simulink model "SMC_controller"  (R2025a)
settings: Solver=VariableStepAuto  StartTime=0.0  StopTime=t_total(end)  RelTol=1e-3
StopFcn:
  | autoplot;
values from neighbouring files (symbols this model uses):
  Ib = diag([params.Ix, params.Iy, params.Iz])    [setup_mission.m]
  lin_vel_0 = [0; 0; 0]    [setup_mission.m]
  mass = params.m    [setup_mission.m]
  pos_0 = p_ref(:,1) + offset_init    [setup_mission.m]
  w_bb_0 = [0; 0; 0]    [setup_mission.m]
libraries: robotcorelib x2, uavutilslib x1
settings Model: Creator=marco  LastModifiedBy=marco

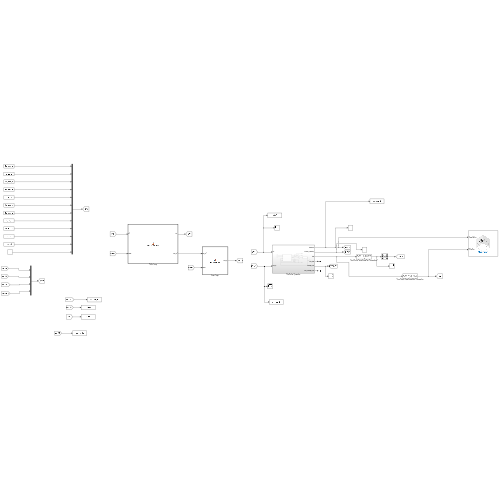
[thumbnail: Simulink's stored preview of the top-level diagram]
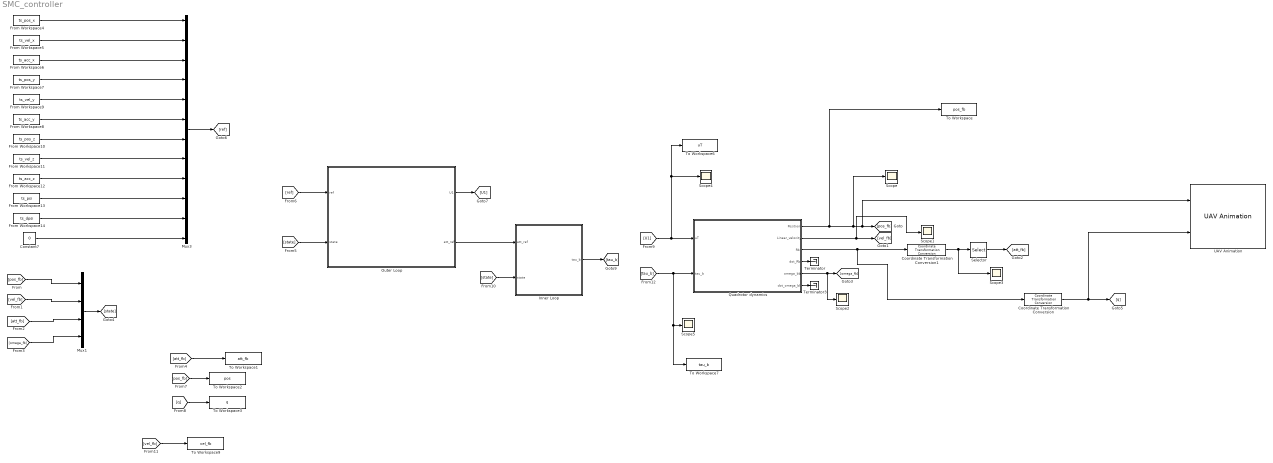
== system SMC_controller ==
  Constant7 : Constant  Value=0
  Coordinate Transformation Conversion : robotcorelib/Coordinate Transformation Conversion  InputRepresentation=Rotation Matrix  InputEulerSequence=ZYX  ShowTrVecInputPort=on  OutputRepresentation=Quaternion  OutputEulerSequence=ZYX  ShowTrVecOutputPort=on  SimulateUsing=Interpreted execution
  Coordinate Transformation Conversion1 : robotcorelib/Coordinate Transformation Conversion  InputRepresentation=Rotation Matrix  InputEulerSequence=ZYX  ShowTrVecInputPort=on  OutputRepresentation=Euler Angles  OutputEulerSequence=ZYX  ShowTrVecOutputPort=on  SimulateUsing=Interpreted execution
  From Workspace10 : FromWorkspace  VariableName=ts_pos_z
  From Workspace11 : FromWorkspace  VariableName=ts_vel_z
  From Workspace12 : FromWorkspace  VariableName=ts_acc_z
  From Workspace13 : FromWorkspace  VariableName=ts_psi
  From Workspace14 : FromWorkspace  VariableName=ts_dpsi
  From Workspace4 : FromWorkspace  VariableName=ts_pos_x
  From Workspace5 : FromWorkspace  VariableName=ts_vel_x
  From Workspace6 : FromWorkspace  VariableName=ts_acc_x
  From Workspace7 : FromWorkspace  VariableName=ts_pos_y
  From Workspace8 : FromWorkspace  VariableName=ts_acc_y
  From Workspace9 : FromWorkspace  VariableName=ts_vel_y
  Inner Loop : MATLAB Function  TreatAsAtomicUnit=on
  Mux1 : Mux
  Mux3 : Mux  Inputs=12
  Outer Loop : MATLAB Function  TreatAsAtomicUnit=on
  Quadrotor dynamics : Subsystem
  Scope{,1..5} (6 alike) : Scope
      Scope settings: ActiveDisplayYMinimum=-3.15015245464377  ActiveDisplayYMaximum=14.919654121534494
      Scope1 settings: ActiveDisplayYMinimum=-2.7455147256808767  ActiveDisplayYMaximum=2.7455147553704635
      Scope2 settings: ActiveDisplayYMinimum=-1  ActiveDisplayYMaximum=1  DataLoggingVariableName=ScopeData2
      Scope3 settings: ActiveDisplayYMinimum=-1  ActiveDisplayYMaximum=1  DataLoggingVariableName=ScopeData3
      Scope4 settings: ActiveDisplayYMinimum=4.05773159000642  ActiveDisplayYMaximum=6.8393308416800735  DataLoggingVariableName=ScopeData4
      Scope5 settings: ActiveDisplayYMinimum=-0.047587391271412371  ActiveDisplayYMaximum=0.017818503987418778  DataLoggingVariableName=ScopeData5
  Selector : Selector  InputPortWidth=3  IndexOptions=Index vector (dialog)  Indices=[3, 2, 1]  OutputSizes=1
  Terminator : Terminator
  Terminator3 : Terminator
  To Workspace : ToWorkspace  VariableName=pos_fb  SaveFormat=Timeseries  SampleTime=-1
  To Workspace1 : ToWorkspace  VariableName=att_fb  SaveFormat=Timeseries  SampleTime=-1
  To Workspace2 : ToWorkspace  VariableName=pos  SaveFormat=Timeseries  SampleTime=-1
  To Workspace3 : ToWorkspace  VariableName=q  SaveFormat=Timeseries  SampleTime=-1
  To Workspace6 : ToWorkspace  VariableName=uT  SaveFormat=Timeseries  SampleTime=-1
  To Workspace7 : ToWorkspace  VariableName=tau_b  SaveFormat=Timeseries  SampleTime=-1
  To Workspace9 : ToWorkspace  VariableName=vel_fb  SaveFormat=Timeseries  SampleTime=-1
  UAV Animation : uavutilslib/UAV Animation  NumUAV=1  DynamicUAVConfig=off  UAVType=Multirotor  UAVSize=1  UAVColor=[1 0 0]  UAVTrajectoryAlpha=1  InertialZDirection=Down  RotationFormat=Quaternion  DrawMarkers=off  SampleTime=0.01
  wires:
  [att_fb] -> Mux1/3
  [pos_fb] -> Mux1/1
  Selector/1 -> [att_fb]
  [omega_fb] -> Mux1/4
  Coordinate Transformation Conversion1/1 -> Selector/1, Scope3/1
  Quadrotor dynamics/3(Rb) -> Coordinate Transformation Conversion/1, Coordinate Transformation Conversion1/1
  Quadrotor dynamics/2(Linear_velocity) -> Scope1/1, [vel_fb]
  Quadrotor dynamics/1(Position) -> To Workspace/1, Scope/1, UAV Animation/1, [pos_fb]
  Quadrotor dynamics/5(omega_bb) -> Scope2/1, [omega_fb]
  Coordinate Transformation Conversion/1 -> UAV Animation/2, [q]
  [vel_fb] -> Mux1/2
  Quadrotor dynamics/4(dot_Rb) -> Terminator/1
  Quadrotor dynamics/6(dot_omega_bb) -> Terminator3/1
  [att_fb] -> To Workspace1/1
  Mux1/1 -> [state]
  Mux3/1 -> [ref]
  From Workspace6/1 -> Mux3/3
  From Workspace5/1 -> Mux3/2
  From Workspace4/1 -> Mux3/1
  From Workspace7/1 -> Mux3/4
  From Workspace9/1 -> Mux3/5
  From Workspace8/1 -> Mux3/6
  From Workspace10/1 -> Mux3/7
  From Workspace11/1 -> Mux3/8
  From Workspace12/1 -> Mux3/9
  From Workspace13/1 -> Mux3/10
  Constant7/1 -> Mux3/12
  From Workspace14/1 -> Mux3/11
  [pos_fb] -> To Workspace2/1
  [q] -> To Workspace3/1
  [vel_fb] -> To Workspace9/1
  [state] -> Inner Loop/2(state)
  Inner Loop/1(tau_b) -> [tau_b]
  Outer Loop/2(att_ref) -> Inner Loop/1(att_ref)
  Outer Loop/1(U1) -> [U1]
  [state] -> Outer Loop/2(state)
  [ref] -> Outer Loop/1(ref)
  [U1] -> Scope4/1, To Workspace6/1, Quadrotor dynamics/1(uT)
  [tau_b] -> To Workspace7/1, Scope5/1, Quadrotor dynamics/2(tau_b)

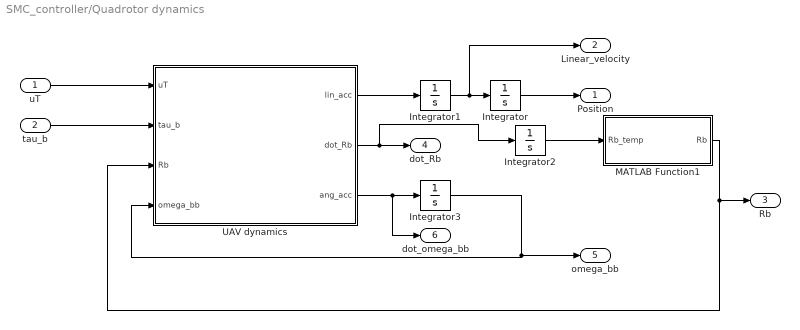
== system SMC_controller/Quadrotor dynamics ==
  uT : Inport
  tau_b : Inport  Port=2
  Integrator : Integrator  InitialCondition=pos_0
  Integrator1 : Integrator  InitialCondition=lin_vel_0
  Integrator2 : Integrator  InitialCondition=[1 0 0; 0 1 0;0 0 1]
  Integrator3 : Integrator  InitialCondition=w_bb_0
  MATLAB Function1 : MATLAB Function  TreatAsAtomicUnit=on
  UAV dynamics : MATLAB Function  TreatAsAtomicUnit=on
  Position : Outport
  Linear_velocity : Outport  Port=2
  Rb : Outport  Port=3
  dot_Rb : Outport  Port=4
  omega_bb : Outport  Port=5
  dot_omega_bb : Outport  Port=6
  wires:
  tau_b/1 -> UAV dynamics/2(tau_b)
  Integrator/1 -> Position/1
  UAV dynamics/3(ang_acc) -> dot_omega_bb/1, Integrator3/1
  UAV dynamics/1(lin_acc) -> Integrator1/1
  uT/1 -> UAV dynamics/1(uT)
  Integrator1/1 -> Linear_velocity/1, Integrator/1
  Integrator3/1 -> UAV dynamics/4(omega_bb), omega_bb/1
  UAV dynamics/2(dot_Rb) -> Integrator2/1, dot_Rb/1
  MATLAB Function1/1(Rb) -> Rb/1, UAV dynamics/3(Rb)
  Integrator2/1 -> MATLAB Function1/1(Rb_temp)

== matlab function SMC_controller/Quadrotor dynamics/UAV dynamics ==
  data: uT input size=1; tau_b input size=3; lin_acc output size=3; Rb input size=[3,3]; omega_bb input size=3; dot_Rb output size=[3,3]; ang_acc output size=3; mass parameter size=1; Ib parameter size=[3,3]
function [lin_acc, dot_Rb, ang_acc] = fcn(uT,tau_b,Rb,omega_bb,mass, Ib)

lin_acc = 9.81*[0 0 1]'-(uT/mass)*Rb*[0 0 1]';
dot_Rb = Rb*skew(omega_bb);
ang_acc = inv(Ib)*(-skew(omega_bb)*Ib*omega_bb + tau_b);

end

function S = skew(v)
if(numel(v)~= 1)
S= [0 -v(3) v(2); 
    v(3) 0 -v(1);
    -v(2) v(1) 0];
else
S= zeros(3);
end
end

== matlab function SMC_controller/Outer Loop ==
  data: ref input; U1 output; state input; att_ref output; params parameter
function [U1, att_ref] = smc_outer_loop(ref, state, params)
% --- SMC OUTER LOOP (POSIZIONE) ---

%% 1. ESTRAZIONE DATI
x = state(1); y = state(2); z = state(3);
vx = state(4); vy = state(5); vz = state(6);
psi = state(9); % Serve per estrarre gli angoli desiderati

xd = ref(1); vxd = ref(2); axd = ref(3);
yd = ref(4); vyd = ref(5); ayd = ref(6);
zd = ref(7); vzd = ref(8); azd = ref(9);
psid = ref(10); dpsid = ref(11);

m = params.m; g = params.g;

%% 2. PARAMETRI DI TUNING (Posizione)
lam_x = 4.0;  K_x = 5.0;   
lam_y = 4.0;  K_y = 3.0;   
lam_z = 5.0;  K_z = 12.0;  
sat_width = 0.5; 

%% 3. CONTROLLO POSIZIONE
ex = xd - x;  edot_x = vxd - vx;
ey = yd - y;  edot_y = vyd - vy;
ez = zd - z;  edot_z = vzd - vz;

Sx = edot_x + lam_x * ex;
Sy = edot_y + lam_y * ey;
Sz = edot_z + lam_z * ez;

Ux = axd + lam_x * edot_x + K_x * tanh(Sx / sat_width);
Uy = ayd + lam_y * edot_y + K_y * tanh(Sy / sat_width);
Uz = azd + lam_z * edot_z + K_z * tanh(Sz / sat_width);

% --- Calcolo U1 (Thrust) ---
total_acc_z = g - Uz; 
U1 = m * sqrt(Ux^2 + Uy^2 + total_acc_z^2);

% Safety Clamp
if U1 > 20 * m * g
    U1 = 20 * m * g; 
end

% --- CALCOLO ANGOLI (FIXED) ---
phi_d_raw   = (Uy * cos(psi) - Ux * sin(psi)) / g; 
theta_d_raw = -1 * (Ux * cos(psi) + Uy * sin(psi)) / g;

phi_d   = max(-0.5, min(0.5, phi_d_raw));
theta_d = max(-0.5, min(0.5, theta_d_raw));

%% 4. OUTPUT VERSO L'INNER LOOP
% Pacchettizziamo i riferimenti di attitudine da passare all'Inner Loop
att_ref = [phi_d; theta_d; psid; dpsid];

end

== matlab function SMC_controller/Inner Loop ==
  data: att_ref input; tau_b output; state input; params parameter
function tau_b  = smc_inner_loop(att_ref, state, params)
% --- SMC INNER LOOP (ATTITUDINE) ---

%% 1. ESTRAZIONE DATI
% Estrazione riferimenti dall'Outer Loop
phi_d = att_ref(1); 
theta_d = att_ref(2);
psid = att_ref(3); 
dpsid = att_ref(4);

phi = state(7); theta = state(8); psi = state(9);
p = state(10); q = state(11); r = state(12);

Ix = params.Ix; Iy = params.Iy; Iz = params.Iz;

%% 2. PARAMETRI DI TUNING (Attitudine)
lam_phi = 15.0;   K_phi = 25.0; 
lam_theta = 15.0; K_theta = 25.0;
lam_psi = 8.0;    K_psi = 10.0;
sat_width = 0.5; 

%% 3. CONTROLLO ATTITUDINE
e_phi   = phi_d - phi;
e_theta = theta_d - theta;
e_psi   = psid - psi;

edot_phi   = 0 - p; 
edot_theta = 0 - q; 
edot_psi   = dpsid - r; 

S_phi   = edot_phi   + lam_phi   * e_phi;
S_theta = edot_theta + lam_theta * e_theta;
S_psi   = edot_psi   + lam_psi   * e_psi;

% --- COPPIE STANDARD ---
U2 = Ix * (lam_phi   * edot_phi   + K_phi   * tanh(S_phi   / sat_width));
U3 = Iy * (lam_theta * edot_theta + K_theta * tanh(S_theta / sat_width));
U4 = Iz * (lam_psi   * edot_psi   + K_psi   * tanh(S_psi   / sat_width));

%% 4. OUTPUT
tau_b = [U2; U3; U4];

end

== matlab function SMC_controller/Quadrotor dynamics/MATLAB Function1 ==
  data: Rb_temp input; Rb output
function Rb = fcn(Rb_temp)
    [U,S,V] = svd(Rb_temp);
    sigma = det(U*V');
    S_ = diag([1 1 sigma]);

    Rb = U*S_*V';
end
